simulink model "Channelizer_AIE_testbench"  (R2021a)
settings: Solver=VariableStepAuto  StartTime=0.0  StopTime=4096  RelTol=1e-3
PostLoadFcn:
  | Channelizer_inputs;
values from neighbouring files (symbols this model uses):
  dft = dft_gen_vectors(TT, FF)    [Channelizer_inputs.m]
undefined symbols (not defined in the file or in its folder): S, vsva2197, xcvc1902
libraries: aieBasic x34, dspsrcs4 x16, aieUtilities x16, vmcUtilities x1
settings Model: Creator=robg  LastModifiedBy=robg

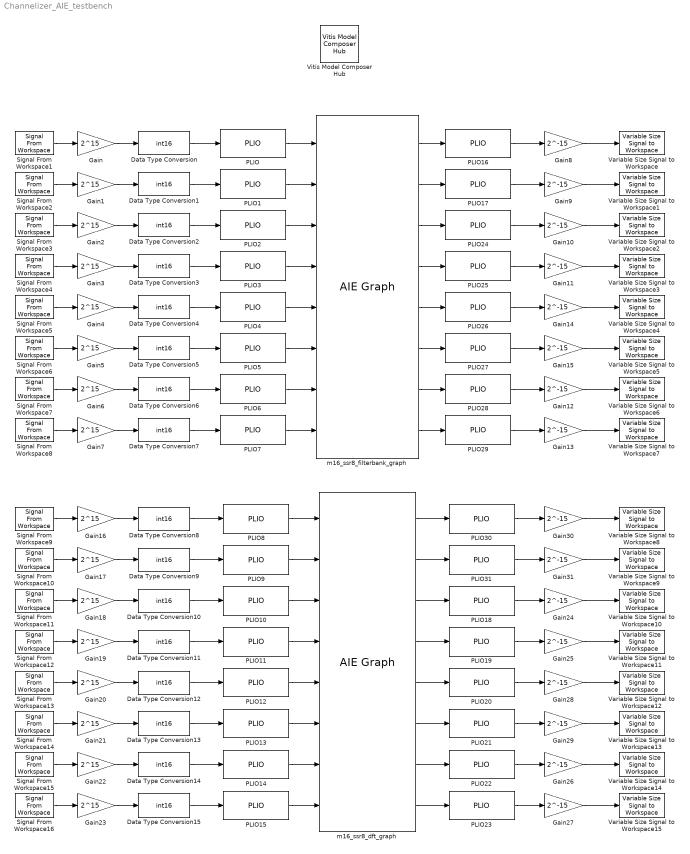
== system Channelizer_AIE_testbench ==
  Data Type Conversion{,1..15} (16 alike) : DataTypeConversion  OutDataTypeStr=int16
  Gain{,1..7,16..23} (16 alike) : Gain  Gain=2^15
  Gain{8..15,24..31} (16 alike) : Gain  Gain=2^-15
  PLIO{,1..31} (32 alike) : aieBasic/PLIO  PlioWidth=128  PlioFreqSpec=off  PlioFreq=250  ColLocation=0  channel=0  blockJsonConstraints=[]  deprecateConstraints=0
  Signal From Workspace1 : dspsrcs4/Signal From Workspace  X=filterbank.sig0_i  Ts=1  nsamps=1  OutputAfterFinalValue=Setting to zero  ignoreOrWarnInputAndFrameLengths=off  OutputFrames=off
  Signal From Workspace10 : dspsrcs4/Signal From Workspace  X=dft(2).i  Ts=1  nsamps=1  OutputAfterFinalValue=Setting to zero  ignoreOrWarnInputAndFrameLengths=off  OutputFrames=off
  Signal From Workspace11 : dspsrcs4/Signal From Workspace  X=dft(7).i  Ts=1  nsamps=1  OutputAfterFinalValue=Setting to zero  ignoreOrWarnInputAndFrameLengths=off  OutputFrames=off
  Signal From Workspace12 : dspsrcs4/Signal From Workspace  X=dft(8).i  Ts=1  nsamps=1  OutputAfterFinalValue=Setting to zero  ignoreOrWarnInputAndFrameLengths=off  OutputFrames=off
  Signal From Workspace13 : dspsrcs4/Signal From Workspace  X=dft(3).i  Ts=1  nsamps=1  OutputAfterFinalValue=Setting to zero  ignoreOrWarnInputAndFrameLengths=off  OutputFrames=off
  Signal From Workspace14 : dspsrcs4/Signal From Workspace  X=dft(4).i  Ts=1  nsamps=1  OutputAfterFinalValue=Setting to zero  ignoreOrWarnInputAndFrameLengths=off  OutputFrames=off
  Signal From Workspace15 : dspsrcs4/Signal From Workspace  X=dft(5).i  Ts=1  nsamps=1  OutputAfterFinalValue=Setting to zero  ignoreOrWarnInputAndFrameLengths=off  OutputFrames=off
  Signal From Workspace16 : dspsrcs4/Signal From Workspace  X=dft(6).i  Ts=1  nsamps=1  OutputAfterFinalValue=Setting to zero  ignoreOrWarnInputAndFrameLengths=off  OutputFrames=off
  Signal From Workspace2 : dspsrcs4/Signal From Workspace  X=filterbank.sig1_i  Ts=1  nsamps=1  OutputAfterFinalValue=Setting to zero  ignoreOrWarnInputAndFrameLengths=off  OutputFrames=off
  Signal From Workspace3 : dspsrcs4/Signal From Workspace  X=filterbank.sig2_i  Ts=1  nsamps=1  OutputAfterFinalValue=Setting to zero  ignoreOrWarnInputAndFrameLengths=off  OutputFrames=off
  Signal From Workspace4 : dspsrcs4/Signal From Workspace  X=filterbank.sig3_i  Ts=1  nsamps=1  OutputAfterFinalValue=Setting to zero  ignoreOrWarnInputAndFrameLengths=off  OutputFrames=off
  Signal From Workspace5 : dspsrcs4/Signal From Workspace  X=filterbank.sig4_i  Ts=1  nsamps=1  OutputAfterFinalValue=Setting to zero  ignoreOrWarnInputAndFrameLengths=off  OutputFrames=off
  Signal From Workspace6 : dspsrcs4/Signal From Workspace  X=filterbank.sig5_i  Ts=1  nsamps=1  OutputAfterFinalValue=Setting to zero  ignoreOrWarnInputAndFrameLengths=off  OutputFrames=off
  Signal From Workspace7 : dspsrcs4/Signal From Workspace  X=filterbank.sig6_i  Ts=1  nsamps=1  OutputAfterFinalValue=Setting to zero  ignoreOrWarnInputAndFrameLengths=off  OutputFrames=off
  Signal From Workspace8 : dspsrcs4/Signal From Workspace  X=filterbank.sig7_i  Ts=1  nsamps=1  OutputAfterFinalValue=Setting to zero  ignoreOrWarnInputAndFrameLengths=off  OutputFrames=off
  Signal From Workspace9 : dspsrcs4/Signal From Workspace  X=dft(1).i  Ts=1  nsamps=1  OutputAfterFinalValue=Setting to zero  ignoreOrWarnInputAndFrameLengths=off  OutputFrames=off
  Variable Size Signal to Workspace : aieUtilities/Variable Size Signal to Workspace  VariableNameMask=filterbank_sig0_o
  Variable Size Signal to Workspace1 : aieUtilities/Variable Size Signal to Workspace  VariableNameMask=filterbank_sig1_o
  Variable Size Signal to Workspace10 : aieUtilities/Variable Size Signal to Workspace  VariableNameMask=dft_sig2_o
  Variable Size Signal to Workspace11 : aieUtilities/Variable Size Signal to Workspace  VariableNameMask=dft_sig3_o
  Variable Size Signal to Workspace12 : aieUtilities/Variable Size Signal to Workspace  VariableNameMask=dft_sig4_o
  Variable Size Signal to Workspace13 : aieUtilities/Variable Size Signal to Workspace  VariableNameMask=dft_sig5_o
  Variable Size Signal to Workspace14 : aieUtilities/Variable Size Signal to Workspace  VariableNameMask=dft_sig6_o
  Variable Size Signal to Workspace15 : aieUtilities/Variable Size Signal to Workspace  VariableNameMask=dft_sig7_o
  Variable Size Signal to Workspace2 : aieUtilities/Variable Size Signal to Workspace  VariableNameMask=filterbank_sig2_o
  Variable Size Signal to Workspace3 : aieUtilities/Variable Size Signal to Workspace  VariableNameMask=filterbank_sig3_o
  Variable Size Signal to Workspace4 : aieUtilities/Variable Size Signal to Workspace  VariableNameMask=filterbank_sig4_o
  Variable Size Signal to Workspace5 : aieUtilities/Variable Size Signal to Workspace  VariableNameMask=filterbank_sig5_o
  Variable Size Signal to Workspace6 : aieUtilities/Variable Size Signal to Workspace  VariableNameMask=filterbank_sig6_o
  Variable Size Signal to Workspace7 : aieUtilities/Variable Size Signal to Workspace  VariableNameMask=filterbank_sig7_o
  Variable Size Signal to Workspace8 : aieUtilities/Variable Size Signal to Workspace  VariableNameMask=dft_sig0_o
  Variable Size Signal to Workspace9 : aieUtilities/Variable Size Signal to Workspace  VariableNameMask=dft_sig1_o
  Vitis Model Composer Hub : vmcUtilities/Vitis Model Composer Hub  Tag=genX  CodeGeneration=off  TargetDirectory=./code  ExportType=AI Engines  IpVendor=xilinx.com  IpLibrary=hls  IpVersion=1.0  IpHWLanguage=Verilog  AieCompilerOptions={}  AieSimulatorOptions={}  CreateTestbench=off  TestbenchStackSize=10  RunAieSim=off  AieSimTimeout=50000  RunAieSimProfiling=off  LaunchVitisAnalyzer=off  PlotOutput=off  RunX86Sim=off  X86SimTimeout=10  GenHwImage=off  PlatformType=Specify Platform  Platform=/proj/xbuilds/SWIP/9999.0_0124_0703/installs/lin64/Vitis/2023.1/base_platforms/xilinx_vck190_base_202310_1/xilinx_vck190_base_202310_1.xpfm  HwSystemType=Baremetal  HwValidationTarget=hw  ProjDevice=Versal VCK190 Evaluation Platform (xcvc1902-vsva2197-2MP-e-S)  ProjDevicePart=xcvc1902-vsva2197-2MP-e-S  SamplePeriod=-1  ClockFrequency=200  DataPathParallelism=1  xilinxfamily=versalaicore  part=xcvc1902  speed=-2MP-e-S  package=vsva2197  directory=./netlist  testbench=off  incr_netlist=off  synthesis_tool=Vivado  clock_wrapper=Clock Enables  dbl_ovrd=According to Block Masks  dcm_input_clock_period=10  sysclk_period=10  simulink_period=1  eval_field=0  LogFileName=''  NThreads=4
  m16_ssr8_dft_graph : aieBasic/AIE Graph  PortAttributesTable={ 'Input', 'sig_i[0]', 'stream', 'cint16', '', '', ''; 'Input', 'sig_i[1]', 'stream', 'cint16', '', '', ''; 'Input', 'sig_i[6]', 'stream', 'cint16', '', '', ''; 'Input', 'sig_i[7]', 'stream', 'cint16', '', '', ''; 'Input', 'sig_i[2]', 'stream', 'cint16', '', '', ''; 'Input', 'sig_i[3]', 'stream', 'cint16', '', '', ''; 'Input', 'sig_i[4]', 'stream', 'cint16', '', '', ''; 'Input', 'sig_i[5]', 'stream', 'cint16', '', '', ''; 'Output', 'sig_o[0]', 'stream', 'cint16', '', '', '1'; 'Output', 'sig_o[1]', 'stream', 'cint16', '', '', '1'; 'Output', 'sig_o[2]', 'stream', 'cint16', '', '', '1'; 'Output', 'sig_o[3]', 'stream', 'cint16', '', '', '1'; 'Output', 'sig_o[4]', 'stream', 'cint16', '', '', '1'; 'Output', 'sig_o[5]', 'stream', 'cint16', '', '', '1'; 'Output', 'sig_o[6]', 'stream', 'cint16', '', '', '1'; 'Output', 'sig_o[7]', 'stream', 'cint16', '', '', '1' }  PortAttributesEnablement={'off', 'on', 'off', 'off', 'off', 'off', 'off';'off', 'on', 'off', 'off', 'off', 'off', 'off';'off', 'on', 'off', 'off', 'off', 'off', 'off';'off', 'on', 'off', 'off', 'off', 'off', 'off';'off', 'on', 'off', 'off', 'off', 'off', 'off';'off', 'on', 'off', 'off', 'off', 'off', 'off';'off', 'on', 'off', 'off', 'off', 'off', 'off';'off', 'on', 'off', 'off', 'off', 'off', 'off';'off', 'on', 'off', 'off', 'off', 'off', 'on';'off', 'on', 'off', 'off', 'off', 'off', 'on';'off', 'on', 'off', 'off', 'off', 'off', 'on';'off', 'on', 'off', 'off', 'off', 'off', 'on';'off', 'on', 'off', 'off', 'off', 'off', 'on';'off', 'on', 'off', 'off', 'off', 'off', 'on';'off', 'on', 'off', 'off', 'off', 'off', 'on';'off', 'on', 'off', 'off', 'off', 'off', 'on'}  SampleTime=-1  ClassDeclTypeOptions=C[1 1]@t24@class m16_ssr8_dft_graph  ClassDecl=class m16_ssr8_dft_graph  ClassTemplateParams={}  ClassTemplateParamsEnables={}  ClassPortParams={ 'input', 'sig_i,8>', 'off'; 'output', 'sig_o,8>', 'off' }  ClassCtorDeclTypeOptions=C[1 1]@t7@<empty>  ClassCtorDecl=<empty>  ClassCtorParams={}  GraphAllAttrs=|  PortArgDecls={'in stream cint16 in1'; 'in stream cint16 in2'; 'in stream cint16 in3'; 'in stream cint16 in4'; 'in stream cint16 in5'; 'in stream cint16 in6'; 'in stream cint16 in7'; 'in stream cint16 in8'; 'out stream cint16 out1'; 'out stream cint16 out2'; 'out stream cint16 out3'; 'out stream cint16 out4'; 'out stream cint16 out5'; 'out stream cint16 out6'; 'out stream cint16 out7'; 'out stream cint16 out8'}  PortGraphPortNames={'sig_i[0]'; 'sig_i[1]'; 'sig_i[6]'; 'sig_i[7]'; 'sig_i[2]'; 'sig_i[3]'; 'sig_i[4]'; 'sig_i[5]'; 'sig_o[0]'; 'sig_o[1]'; 'sig_o[2]'; 'sig_o[3]'; 'sig_o[4]'; 'sig_o[5]'; 'sig_o[6]'; 'sig_o[7]'}  PortTypes={'stream'; 'stream'; 'stream'; 'stream'; 'stream'; 'stream'; 'stream'; 'stream'; 'stream'; 'stream'; 'stream'; 'stream'; 'stream'; 'stream'; 'stream'; 'stream'}  PortDataTypes={'cint16'; 'cint16'; 'cint16'; 'cint16'; 'cint16'; 'cint16'; 'cint16'; 'cint16'; 'cint16'; 'cint16'; 'cint16'; 'cint16'; 'cint16'; 'cint16'; 'cint16'; 'cint16'}  PortSizes={0.000000000000000000e+00; 0.000000000000000000e+00; 0.000000000000000000e+00; 0.000000000000000000e+00; 0.000000000000000000e+00; 0.000000000000000000e+00; 0.000000000000000000e+00; 0.000000000000000000e+00; 0.000000000000000000e+00; 0.000000000000000000e+00; 0.000000000000000000e+00; 0.000000000000000000e+00; 0.000000000000000000e+00; 0.000000000000000000e+00; 0.000000000000000000e+00; 0.000000000000000000e+00}  PortSynchronicities={'auto'; 'auto'; 'auto'; 'auto'; 'auto'; 'auto'; 'auto'; 'auto'; 'auto'; 'auto'; 'auto'; 'auto'; 'auto'; 'auto'; 'auto'; 'auto'}  PortSignalSizes={0.000000000000000000e+00; 0.000000000000000000e+00; 0.000000000000000000e+00; 0.000000000000000000e+00; 0.000000000000000000e+00; 0.000000000000000000e+00; 0.000000000000000000e+00; 0.000000000000000000e+00; 1.000000000000000000e+00; 1.000000000000000000e+00; 1.000000000000000000e+00; 1.000000000000000000e+00; 1.000000000000000000e+00; 1.000000000000000000e+00; 1.000000000000000000e+00; 1.000000000000000000e+00}  SimLibPath=''  ClassIndex=1  ClassCtorIndex=0  ClassTabVisible=off  FunctionTabVisible=on  DelayDrawLabels=off  GraphFileSelect=Header file (*.h)  GraphHeaderFile=/proj/xcoswmktg/robg/git/designs/channelizer/aie/m16_ssr8_dft/m16_ssr8_dft_graph.h  GraphClassName=m16_ssr8_dft_graph  GraphName=m16_ssr8_dft_graph  GraphHeaderFiles={'/proj/xcoswmktg/robg/git/designs/channelizer/aie/m16_ssr8_dft/dft_1xN_widget_graph.h'; '/proj/xcoswmktg/robg/git/designs/channelizer/aie/m16_ssr8_dft/m16_ssr8_dft_graph.h'}  GraphSourceFile=./model_composer_work/xmc_aie_lib/8d40d72d/mygraph.cpp  GraphSearchPaths={'/proj/xcoswmktg/robg/git/designs/channelizer/aie/m16_ssr8_dft'}  GraphPreProcOptions={}  blockJsonConstraints=[]  deprecateConstraints=0
      | s[12;12;9;9;19;14;21;23;21;23;24;21;15;17;12;24;26;26;26;27;28;9;21;23;23;23;24;25;14;19;19;29]@FunctionNameDeclFileNamePortNamesPortTypesPortSerializedTypesPortDirectionsPortWindowSizeEnablesPortWindowMarginEnablesPortBufferSizeEnablesPortBufferMarginEnablesPortSynchronicityEnablesPortSignalSizeEnablesPortBufferSizesPortBufferMarginsFunctionDeclFunctionTemplateSpecKindFunctionTemplateParamNamesFunctionTemplateParamKindsFunctionTemplateParamTypesFunctionTemplateParamValuesFunctionTemplateParamEnablesClassDeclClassTemplateSpecKindClassTemplateParamNamesClassTemplateParamKindsClassTemplateParamTypesClassTemplateParamValuesClassTemplateParamEnablesClassCtorDeclsClassCtorParamNamesClassCtorParamTypesClassCtorParamSerializedTypes[1 1]@C[32 1]@nt82@/proj/xcoswmktg/robg/git/designs/channelizer/aie/m16_ssr8_dft/m16_ssr8_dft_graph.hC[2 1]@t5@sig_it5@sig_oC[2 1]@t48@std::array< adf::port< adf::direction::in >, 8 >t49@std::array< adf::port< adf::direction::out >, 8 >C[2 1]@t64@{Tstd::array{2{t{Tadf::port{1{t{Sadf::direction::in}}}}}{t{}8}}}t65@{Tstd::array{2{t{Tadf::port{1{t{Sadf::direction::out}}}}}{t{}8}}}C[2 1]@t5@inputt5@inputC[2 1]@l0@l0@C[2 1]@l0@l0@C[2 1]@l0@l0@C[2 1]@l0@l0@C[2 1]@l1@l1@C[2 1]@l0@l0@C[2 1]@nnC[2 1]@nnt139@void m16_ssr8_dft_graph::
      | (std::array< adf::port< adf::direction::in >, 8 > sig_i, std::array< adf::port< adf::direction::out >, 8 > sig_o)ne[0 1]@e[0 1]@e[0 1]@e[0 1]@e[0 1]@t25@class m16_ssr8_dft_graph;t4@nonee[0 1]@e[0 1]@e[0 1]@e[0 1]@e[0 1]@e[0 1]@e[0 1]@e[0 1]@e[0 1]@
  m16_ssr8_filterbank_graph : aieBasic/AIE Graph  PortAttributesTable={ 'Input', 'sig_i[0]', 'stream', 'cint16', '', '', ''; 'Input', 'sig_i[1]', 'stream', 'cint16', '', '', ''; 'Input', 'sig_i[2]', 'stream', 'cint16', '', '', ''; 'Input', 'sig_i[3]', 'stream', 'cint16', '', '', ''; 'Input', 'sig_i[4]', 'stream', 'cint16', '', '', ''; 'Input', 'sig_i[5]', 'stream', 'cint16', '', '', ''; 'Input', 'sig_i[6]', 'stream', 'cint16', '', '', ''; 'Input', 'sig_i[7]', 'stream', 'cint16', '', '', ''; 'Output', 'sig_o[0]', 'stream', 'cint16', '', '', '1'; 'Output', 'sig_o[1]', 'stream', 'cint16', '', '', '1'; 'Output', 'sig_o[2]', 'stream', 'cint16', '', '', '1'; 'Output', 'sig_o[3]', 'stream', 'cint16', '', '', '1'; 'Output', 'sig_o[4]', 'stream', 'cint16', '', '', '1'; 'Output', 'sig_o[5]', 'stream', 'cint16', '', '', '1'; 'Output', 'sig_o[6]', 'stream', 'cint16', '', '', '1'; 'Output', 'sig_o[7]', 'stream', 'cint16', '', '', '1' }  PortAttributesEnablement={'off', 'on', 'off', 'off', 'off', 'off', 'off';'off', 'on', 'off', 'off', 'off', 'off', 'off';'off', 'on', 'off', 'off', 'off', 'off', 'off';'off', 'on', 'off', 'off', 'off', 'off', 'off';'off', 'on', 'off', 'off', 'off', 'off', 'off';'off', 'on', 'off', 'off', 'off', 'off', 'off';'off', 'on', 'off', 'off', 'off', 'off', 'off';'off', 'on', 'off', 'off', 'off', 'off', 'off';'off', 'on', 'off', 'off', 'off', 'off', 'on';'off', 'on', 'off', 'off', 'off', 'off', 'on';'off', 'on', 'off', 'off', 'off', 'off', 'on';'off', 'on', 'off', 'off', 'off', 'off', 'on';'off', 'on', 'off', 'off', 'off', 'off', 'on';'off', 'on', 'off', 'off', 'off', 'off', 'on';'off', 'on', 'off', 'off', 'off', 'off', 'on';'off', 'on', 'off', 'off', 'off', 'off', 'on'}  SampleTime=-1  ClassDeclTypeOptions=C[1 1]@t31@class m16_ssr8_filterbank_graph  ClassDecl=class m16_ssr8_filterbank_graph  ClassTemplateParams={}  ClassTemplateParamsEnables={}  ClassPortParams={ 'input', 'sig_i,8>', 'off'; 'output', 'sig_o,8>', 'off' }  ClassCtorDeclTypeOptions=C[1 1]@t7@<empty>  ClassCtorDecl=<empty>  ClassCtorParams={}  GraphAllAttrs=|  PortArgDecls={'in stream cint16 in1'; 'in stream cint16 in2'; 'in stream cint16 in3'; 'in stream cint16 in4'; 'in stream cint16 in5'; 'in stream cint16 in6'; 'in stream cint16 in7'; 'in stream cint16 in8'; 'out stream cint16 out1'; 'out stream cint16 out2'; 'out stream cint16 out3'; 'out stream cint16 out4'; 'out stream cint16 out5'; 'out stream cint16 out6'; 'out stream cint16 out7'; 'out stream cint16 out8'}  PortGraphPortNames={'sig_i[0]'; 'sig_i[1]'; 'sig_i[2]'; 'sig_i[3]'; 'sig_i[4]'; 'sig_i[5]'; 'sig_i[6]'; 'sig_i[7]'; 'sig_o[0]'; 'sig_o[1]'; 'sig_o[2]'; 'sig_o[3]'; 'sig_o[4]'; 'sig_o[5]'; 'sig_o[6]'; 'sig_o[7]'}  PortTypes={'stream'; 'stream'; 'stream'; 'stream'; 'stream'; 'stream'; 'stream'; 'stream'; 'stream'; 'stream'; 'stream'; 'stream'; 'stream'; 'stream'; 'stream'; 'stream'}  PortDataTypes={'cint16'; 'cint16'; 'cint16'; 'cint16'; 'cint16'; 'cint16'; 'cint16'; 'cint16'; 'cint16'; 'cint16'; 'cint16'; 'cint16'; 'cint16'; 'cint16'; 'cint16'; 'cint16'}  PortSizes={0.000000000000000000e+00; 0.000000000000000000e+00; 0.000000000000000000e+00; 0.000000000000000000e+00; 0.000000000000000000e+00; 0.000000000000000000e+00; 0.000000000000000000e+00; 0.000000000000000000e+00; 0.000000000000000000e+00; 0.000000000000000000e+00; 0.000000000000000000e+00; 0.000000000000000000e+00; 0.000000000000000000e+00; 0.000000000000000000e+00; 0.000000000000000000e+00; 0.000000000000000000e+00}  PortSynchronicities={'auto'; 'auto'; 'auto'; 'auto'; 'auto'; 'auto'; 'auto'; 'auto'; 'auto'; 'auto'; 'auto'; 'auto'; 'auto'; 'auto'; 'auto'; 'auto'}  PortSignalSizes={0.000000000000000000e+00; 0.000000000000000000e+00; 0.000000000000000000e+00; 0.000000000000000000e+00; 0.000000000000000000e+00; 0.000000000000000000e+00; 0.000000000000000000e+00; 0.000000000000000000e+00; 1.000000000000000000e+00; 1.000000000000000000e+00; 1.000000000000000000e+00; 1.000000000000000000e+00; 1.000000000000000000e+00; 1.000000000000000000e+00; 1.000000000000000000e+00; 1.000000000000000000e+00}  SimLibPath=''  ClassIndex=1  ClassCtorIndex=0  ClassTabVisible=off  FunctionTabVisible=on  DelayDrawLabels=off  GraphFileSelect=Header file (*.h)  GraphHeaderFile=/proj/xcoswmktg/robg/git/designs/channelizer/aie/m16_ssr8_filterbank/m16_ssr8_filterbank_graph.h  GraphClassName=m16_ssr8_filterbank_graph  GraphName=m16_ssr8_filterbank_graph  GraphHeaderFiles={'/proj/xcoswmktg/robg/git/designs/channelizer/aie/m16_ssr8_filterbank/polyphase_fir_graph.h'; '/proj/xcoswmktg/robg/git/designs/channelizer/aie/m16_ssr8_filterbank/m16_ssr8_filterbank_graph.h'}  GraphSourceFile=./model_composer_work/xmc_aie_lib/fadd8e47/mygraph.cpp  GraphSearchPaths={'/proj/xcoswmktg/robg/git/designs/channelizer/aie/m16_ssr8', '/proj/xcoswmktg/robg/git/designs/channelizer/aie/m16_ssr8_dft', '/proj/xcoswmktg/robg/git/designs/channelizer/aie/m16_ssr8_filterbank'}  GraphPreProcOptions={}  blockJsonConstraints=[]  deprecateConstraints=0
      | s[12;12;9;9;19;14;21;23;21;23;24;21;15;17;12;24;26;26;26;27;28;9;21;23;23;23;24;25;14;19;19;29]@FunctionNameDeclFileNamePortNamesPortTypesPortSerializedTypesPortDirectionsPortWindowSizeEnablesPortWindowMarginEnablesPortBufferSizeEnablesPortBufferMarginEnablesPortSynchronicityEnablesPortSignalSizeEnablesPortBufferSizesPortBufferMarginsFunctionDeclFunctionTemplateSpecKindFunctionTemplateParamNamesFunctionTemplateParamKindsFunctionTemplateParamTypesFunctionTemplateParamValuesFunctionTemplateParamEnablesClassDeclClassTemplateSpecKindClassTemplateParamNamesClassTemplateParamKindsClassTemplateParamTypesClassTemplateParamValuesClassTemplateParamEnablesClassCtorDeclsClassCtorParamNamesClassCtorParamTypesClassCtorParamSerializedTypes[1 1]@C[32 1]@nt96@/proj/xcoswmktg/robg/git/designs/channelizer/aie/m16_ssr8_filterbank/m16_ssr8_filterbank_graph.hC[2 1]@t5@sig_it5@sig_oC[2 1]@t48@std::array< adf::port< adf::direction::in >, 8 >t49@std::array< adf::port< adf::direction::out >, 8 >C[2 1]@t64@{Tstd::array{2{t{Tadf::port{1{t{Sadf::direction::in}}}}}{t{}8}}}t65@{Tstd::array{2{t{Tadf::port{1{t{Sadf::direction::out}}}}}{t{}8}}}C[2 1]@t5@inputt5@inputC[2 1]@l0@l0@C[2 1]@l0@l0@C[2 1]@l0@l0@C[2 1]@l0@l0@C[2 1]@l1@l1@C[2 1]@l0@l0@C[2 1]@nnC[2 1]@nnt146@void m16_ssr8_filterbank_graph::
      | (std::array< adf::port< adf::direction::in >, 8 > sig_i, std::array< adf::port< adf::direction::out >, 8 > sig_o)ne[0 1]@e[0 1]@e[0 1]@e[0 1]@e[0 1]@t32@class m16_ssr8_filterbank_graph;t4@nonee[0 1]@e[0 1]@e[0 1]@e[0 1]@e[0 1]@e[0 1]@e[0 1]@e[0 1]@e[0 1]@
  wires:
  PLIO19/1 -> Gain25/1
  Gain24/1 -> Variable Size Signal to Workspace10/1
  Signal From Workspace1/1 -> Gain/1
  Gain15/1 -> Variable Size Signal to Workspace5/1
  Data Type Conversion2/1 -> PLIO2/1
  Signal From Workspace4/1 -> Gain3/1
  m16_ssr8_filterbank_graph/1 -> PLIO16/1
  PLIO15/1 -> m16_ssr8_dft_graph/8
  Signal From Workspace10/1 -> Gain17/1
  Gain5/1 -> Data Type Conversion5/1
  Signal From Workspace5/1 -> Gain4/1
  Gain19/1 -> Data Type Conversion11/1
  m16_ssr8_dft_graph/5 -> PLIO20/1
  Gain17/1 -> Data Type Conversion9/1
  Gain/1 -> Data Type Conversion/1
  Gain22/1 -> Data Type Conversion14/1
  Gain18/1 -> Data Type Conversion10/1
  Signal From Workspace3/1 -> Gain2/1
  PLIO26/1 -> Gain14/1
  PLIO27/1 -> Gain15/1
  PLIO28/1 -> Gain12/1
  m16_ssr8_filterbank_graph/6 -> PLIO27/1
  Gain11/1 -> Variable Size Signal to Workspace3/1
  PLIO24/1 -> Gain10/1
  Signal From Workspace11/1 -> Gain18/1
  PLIO4/1 -> m16_ssr8_filterbank_graph/5
  Gain29/1 -> Variable Size Signal to Workspace13/1
  Gain9/1 -> Variable Size Signal to Workspace1/1
  Signal From Workspace15/1 -> Gain22/1
  PLIO9/1 -> m16_ssr8_dft_graph/2
  Signal From Workspace8/1 -> Gain7/1
  Gain31/1 -> Variable Size Signal to Workspace9/1
  m16_ssr8_filterbank_graph/3 -> PLIO24/1
  Data Type Conversion/1 -> PLIO/1
  Data Type Conversion14/1 -> PLIO14/1
  PLIO16/1 -> Gain8/1
  PLIO8/1 -> m16_ssr8_dft_graph/1
  Gain1/1 -> Data Type Conversion1/1
  m16_ssr8_dft_graph/3 -> PLIO18/1
  PLIO23/1 -> Gain27/1
  m16_ssr8_filterbank_graph/5 -> PLIO26/1
  m16_ssr8_filterbank_graph/4 -> PLIO25/1
  m16_ssr8_filterbank_graph/2 -> PLIO17/1
  Gain26/1 -> Variable Size Signal to Workspace14/1
  PLIO12/1 -> m16_ssr8_dft_graph/5
  PLIO13/1 -> m16_ssr8_dft_graph/6
  Data Type Conversion3/1 -> PLIO3/1
  PLIO6/1 -> m16_ssr8_filterbank_graph/7
  Gain6/1 -> Data Type Conversion6/1
  Signal From Workspace16/1 -> Gain23/1
  PLIO10/1 -> m16_ssr8_dft_graph/3
  Gain13/1 -> Variable Size Signal to Workspace7/1
  PLIO17/1 -> Gain9/1
  Data Type Conversion11/1 -> PLIO11/1
  Gain23/1 -> Data Type Conversion15/1
  Signal From Workspace7/1 -> Gain6/1
  m16_ssr8_dft_graph/7 -> PLIO22/1
  PLIO3/1 -> m16_ssr8_filterbank_graph/4
  PLIO20/1 -> Gain28/1
  PLIO/1 -> m16_ssr8_filterbank_graph/1
  Gain4/1 -> Data Type Conversion4/1
  Signal From Workspace14/1 -> Gain21/1
  m16_ssr8_dft_graph/4 -> PLIO19/1
  PLIO7/1 -> m16_ssr8_filterbank_graph/8
  Gain28/1 -> Variable Size Signal to Workspace12/1
  Gain8/1 -> Variable Size Signal to Workspace/1
  m16_ssr8_dft_graph/1 -> PLIO30/1
  PLIO1/1 -> m16_ssr8_filterbank_graph/2
  PLIO29/1 -> Gain13/1
  Gain14/1 -> Variable Size Signal to Workspace4/1
  Data Type Conversion7/1 -> PLIO7/1
  Gain12/1 -> Variable Size Signal to Workspace6/1
  PLIO31/1 -> Gain31/1
  Signal From Workspace2/1 -> Gain1/1
  PLIO18/1 -> Gain24/1
  Gain20/1 -> Data Type Conversion12/1
  Data Type Conversion1/1 -> PLIO1/1
  Gain16/1 -> Data Type Conversion8/1
  Gain21/1 -> Data Type Conversion13/1
  Data Type Conversion5/1 -> PLIO5/1
  m16_ssr8_dft_graph/8 -> PLIO23/1
  PLIO30/1 -> Gain30/1
  Data Type Conversion8/1 -> PLIO8/1
  Gain2/1 -> Data Type Conversion2/1
  Data Type Conversion12/1 -> PLIO12/1
  Signal From Workspace12/1 -> Gain19/1
  Gain3/1 -> Data Type Conversion3/1
  Data Type Conversion4/1 -> PLIO4/1
  Data Type Conversion15/1 -> PLIO15/1
  Gain30/1 -> Variable Size Signal to Workspace8/1
  PLIO25/1 -> Gain11/1
  Data Type Conversion9/1 -> PLIO9/1
  m16_ssr8_dft_graph/6 -> PLIO21/1
  Signal From Workspace6/1 -> Gain5/1
  Gain7/1 -> Data Type Conversion7/1
  m16_ssr8_filterbank_graph/7 -> PLIO28/1
  Data Type Conversion13/1 -> PLIO13/1
  PLIO14/1 -> m16_ssr8_dft_graph/7
  PLIO2/1 -> m16_ssr8_filterbank_graph/3
  Signal From Workspace13/1 -> Gain20/1
  Gain10/1 -> Variable Size Signal to Workspace2/1
  m16_ssr8_dft_graph/2 -> PLIO31/1
  m16_ssr8_filterbank_graph/8 -> PLIO29/1
  PLIO22/1 -> Gain26/1
  Data Type Conversion10/1 -> PLIO10/1
  PLIO11/1 -> m16_ssr8_dft_graph/4
  PLIO5/1 -> m16_ssr8_filterbank_graph/6
  PLIO21/1 -> Gain29/1
  Data Type Conversion6/1 -> PLIO6/1
  Gain25/1 -> Variable Size Signal to Workspace11/1
  Gain27/1 -> Variable Size Signal to Workspace15/1
  Signal From Workspace9/1 -> Gain16/1
